simulink model "tank_nur_2_punkt"  (R2018b)
settings: Solver=VariableStepAuto  StartTime=0.0  StopTime=100  RelTol=1e-3
settings Model: Creator=Duc  LastModifiedBy=Duc

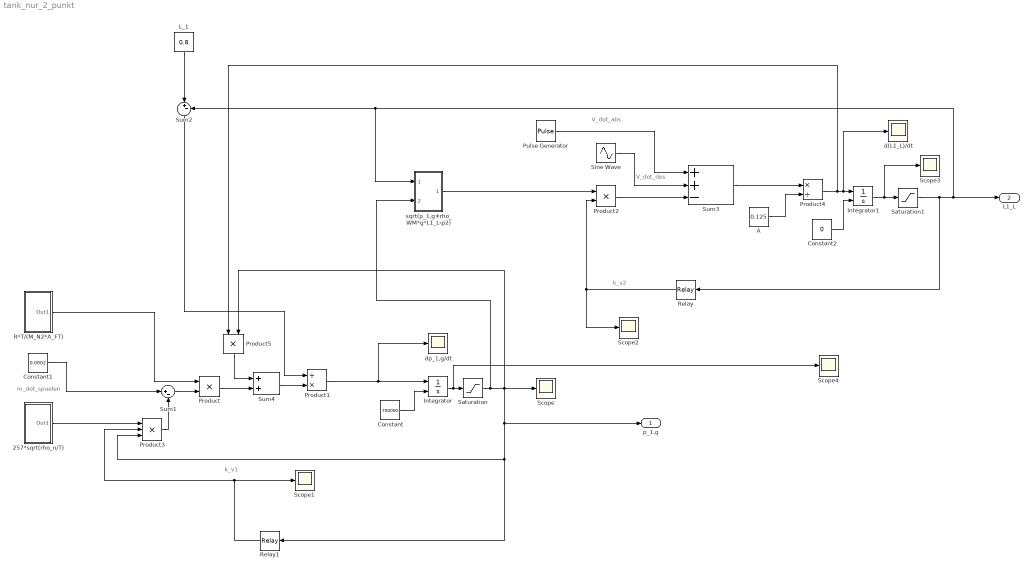
== system tank_nur_2_punkt ==
  note: V_dot_des
  note: V_dot_abs
  note: m_dot_spuelen
  note: k_v1
  note: k_v2
  257*sqrt(rho_n/T) : Subsystem
  A : Constant  Value=0.125
  Constant : Constant  Value=700000
  Constant1 : Constant  Value=0.0002
  Constant2 : Constant  Value=0
  Integrator : Integrator  InitialConditionSource=external  LowerSaturationLimit=0
  Integrator1 : Integrator  InitialConditionSource=external  LowerSaturationLimit=0
  L_1 : Constant  Value=0.8
  Product : Product
  Product1 : Product  Inputs=/*
  Product2 : Product
  Product3 : Product  Inputs=3
  Product4 : Product  Inputs=*/
  Product5 : Product
  Pulse Generator : DiscretePulseGenerator  PulseType=Time based  Amplitude=0.02  Period=5  PulseWidth=5
  R*T/(M_N2*A_FT) : Subsystem
  Relay : Relay  OnSwitchValue=0.6  OffSwitchValue=0.4  OnOutputValue=0.08
  Relay1 : Relay  OnSwitchValue=750000  OffSwitchValue=650000  OnOutputValue=0.00002
  Saturation : Saturate  UpperLimit=3000000  LowerLimit=101325
  Saturation1 : Saturate  UpperLimit=0.79  LowerLimit=0
  Scope{,1..4} (5 alike) : Scope
  Sine Wave : Sin  Amplitude=0.01  Bias=0.01  Frequency=2  SampleTime=0
  Sum1 : Sum  Inputs=|+-
  Sum2 : Sum  Inputs=|+-
  Sum3 : Sum  Inputs=++-
  Sum4 : Sum
  d(L1_L)/dt : Scope
  dp_1,g/dt : Scope
  sqrt(p_1,g+rho_WM*g*L1_L-p2) : Subsystem
  p_1,g : Outport
  L1_L : Outport  Port=2
  wires:
  Relay1/1 -> Scope1/1, Product3/2
  R*T/(M_N2*A_FT)/1(Out1) -> Product/1
  Product1/1 -> Integrator/1, dp_1,g/dt/1
  Sum4/1 -> Product1/2
  Saturation1/1 -> Relay/1, Sum2/2, sqrt(p_1,g+rho_WM*g*L1_L-p2)/1(In1), L1_L/1
  Sum1/1 -> Product/2
  Sum3/1 -> Product4/1
  Sum2/1 -> Product1/1
  Relay/1 -> Scope2/1, Product2/2
  Product5/1 -> Sum4/1
  Product3/1 -> Sum1/2
  Constant/1 -> Integrator/2
  Integrator1/1 -> Saturation1/1, Scope3/1
  L_1/1 -> Sum2/1
  257*sqrt(rho_n/T)/1(Out1) -> Product3/1
  Product/1 -> Sum4/2
  Integrator/1 -> Scope4/1, Saturation/1
  sqrt(p_1,g+rho_WM*g*L1_L-p2)/1(Out1) -> Product2/1
  Constant2/1 -> Integrator1/2
  Saturation/1 -> Product3/3, Relay1/1, p_1,g/1, Scope/1, Product5/2, sqrt(p_1,g+rho_WM*g*L1_L-p2)/2(In2)
  Product2/1 -> Sum3/3
  Sine Wave/1 -> Sum3/2
  A/1 -> Product4/2
  Pulse Generator/1 -> Sum3/1
  Constant1/1 -> Sum1/1
  Product4/1 -> Product5/1, d(L1_L)/dt/1, Integrator1/1

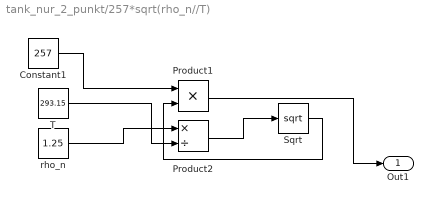
== system tank_nur_2_punkt/257*sqrt(rho_n//T) ==
  Constant1 : Constant  Value=257
  Product1 : Product
  Product2 : Product  Inputs=*/
  Sqrt : Sqrt  SaturateOnIntegerOverflow=on
  T : Constant  Value=293.15
  rho_n : Constant  Value=1.25
  Out1 : Outport
  wires:
  Product2/1 -> Sqrt/1
  Product1/1 -> Out1/1
  Constant1/1 -> Product1/1
  T/1 -> Product2/2
  rho_n/1 -> Product2/1
  Sqrt/1 -> Product1/2

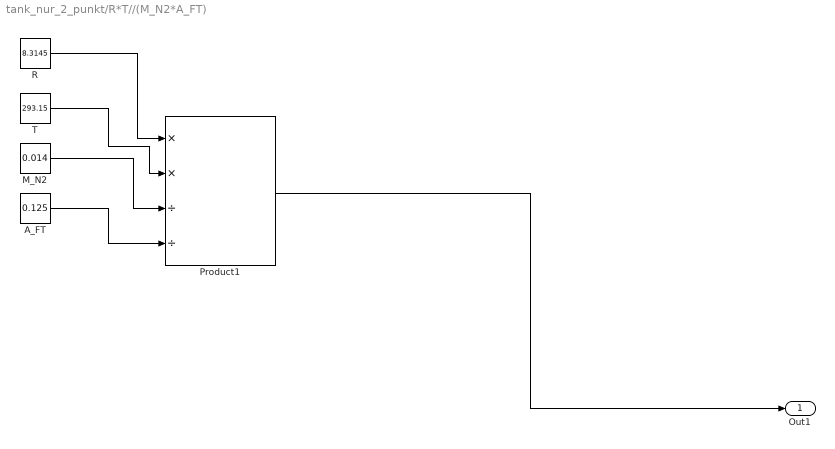
== system tank_nur_2_punkt/R*T//(M_N2*A_FT) ==
  A_FT : Constant  Value=0.125
  M_N2 : Constant  Value=0.014
  Product1 : Product  Inputs=**//
  R : Constant  Value=8.3145
  T : Constant  Value=293.15
  Out1 : Outport
  wires:
  A_FT/1 -> Product1/4
  Product1/1 -> Out1/1
  T/1 -> Product1/2
  R/1 -> Product1/1
  M_N2/1 -> Product1/3

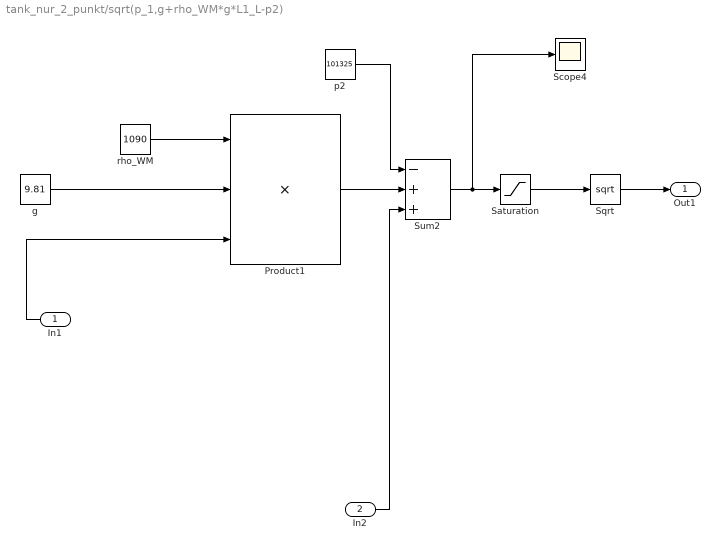
== system tank_nur_2_punkt/sqrt(p_1,g+rho_WM*g*L1_L-p2) ==
  In1 : Inport
  In2 : Inport  Port=2
  Product1 : Product  Inputs=***
  Saturation : Saturate  UpperLimit=inf  LowerLimit=0
  Scope4 : Scope
  Sqrt : Sqrt  SaturateOnIntegerOverflow=on
  Sum2 : Sum  Inputs=-++
  g : Constant  Value=9.81
  p2 : Constant  Value=101325
  rho_WM : Constant  Value=1090
  Out1 : Outport
  wires:
  rho_WM/1 -> Product1/1
  Product1/1 -> Sum2/2
  g/1 -> Product1/2
  In1/1 -> Product1/3
  Sqrt/1 -> Out1/1
  p2/1 -> Sum2/1
  In2/1 -> Sum2/3
  Sum2/1 -> Scope4/1, Saturation/1
  Saturation/1 -> Sqrt/1
